simulink model "VV_MPC"  (R2017a)
settings: Solver=VariableStepAuto  StartTime=0.0  StopTime=0.5  RelTol=1e-3
values from neighbouring files (symbols this model uses):
  X = fsolve(@(x)VanVusseModel(t,x,u,k10,k20,k30,E1,E2,E3,deltaAB,deltaBC,deltaAD,ro,cp,Kw,Ar,Ca0,T0,V),x0)    [mainVV.m]
libraries: mpclib x1
settings Model: Creator=Sergio  LastModifiedBy=Sergio

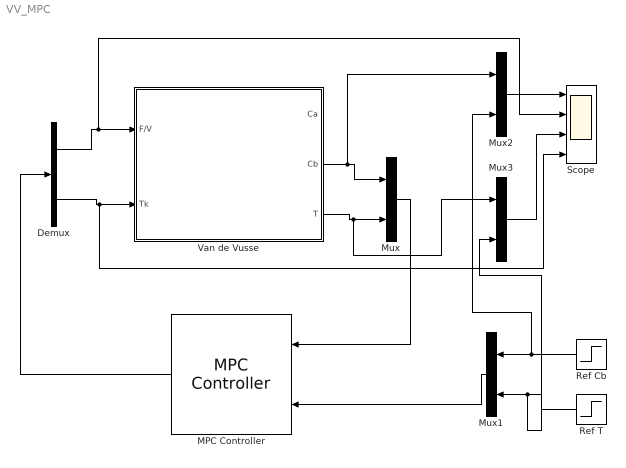
== system VV_MPC ==
  Demux : Demux  Outputs=2
  MPC Controller : mpclib/MPC Controller  SCDEnableBlockLinearizationSpecification=on  mpcobj=mpc1  is_multiple=0  enable_value=0  return_u0=off  ref_from_ws=off  ref_signal_name=[]  ref_preview=off  md_from_ws=off  md_signal_name=[]  md_preview=off  from_project=off  project_file=MPCtask.mat  md_inport=off  mv_inport=off  cost_outport=off  return_sequence=off  return_qpstatus=off  return_state=off  state_inport=off  lims_inport=off  ywt_inport=off  is_designfromscratch=0  uwt_inport=off  duwt_inport=off  rhoeps_inport=off  uref_inport=off  n_ts=0.005  n_mv=2  n_md=0  n_ud=0  n_mo=2  n_uo=0  BlockDataType=double  SampleTimeInherited=off  switch_inport=off
  Mux{,1..3} (4 alike) : Mux  Inputs=2
  Ref Cb : Step  Time=0.1  Before=X(2)  After=X(2)-0.1  SampleTime=0
  Ref T : Step  Time=0.3  Before=X(3)  After=X(3)-6  SampleTime=0
  Scope : Scope  NumInputPorts=4
  Van de Vusse : Subsystem
      mask Display: image('C:\Users\Sergio\Dropbox\UFRJ\DINÂMICA E CONTROLE DE PROCESSOS\Trabalho3\Codigos\VanVUsse.png');
  wires:
  Mux2/1 -> Scope/1
  Ref T/1 -> Mux3/2, Mux1/2
  Ref Cb/1 -> Mux2/2, Mux1/1
  Van de Vusse/3(T) -> Mux3/1, Mux/2
  MPC Controller/1 -> Demux/1
  Demux/1 -> Scope/2, Van de Vusse/1(F/V)
  Mux3/1 -> Scope/3
  Mux1/1 -> MPC Controller/2
  Van de Vusse/2(Cb) -> Mux2/1, Mux/1
  Mux/1 -> MPC Controller/1
  Demux/2 -> Scope/4, Van de Vusse/2(Tk)

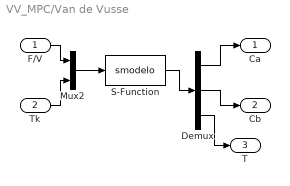
== system VV_MPC/Van de Vusse ==
  F/V : Inport
  Tk : Inport  Port=2
  Demux : Demux  Outputs=3
  Mux2 : Mux  Inputs=2
  S-Function : S-Function  FunctionName=smodelo  Parameters="1.287e12,1.287e12,9.043e9, -9758.3, -9758.3, -8560.0, -4.2, 11.0, 41.85, 0.9342, 3.01, 4032.0, 0.215, 5.1, 130.0, 10, 2.4499,    1.1033,  136.7606"  SFunctionDeploymentMode=off  EnableBusSupport=off
  Ca : Outport
  Cb : Outport  Port=2
  T : Outport  Port=3
  wires:
  Demux/3 -> T/1
  F/V/1 -> Mux2/1
  Demux/2 -> Cb/1
  Tk/1 -> Mux2/2
  Demux/1 -> Ca/1
  S-Function/1 -> Demux/1
  Mux2/1 -> S-Function/1
